simulink model "building_EXAMPLE_v1"  (R2016b)
settings: Solver=ode23tb  StartTime=-building.preruntime+8760*3600  StopTime=building.runtime+8760*3600  MaxStep=600  EnableMultiTasking=on
StartFcn:
  | tic
StopFcn:
  | toc
values from neighbouring files (symbols this model uses):
  building = create_building_automatic(building, modify, import_mode, name_XML, name_EXCEL, name_PHPP, NUMBEROFZONES)    [work_EXAMPLE_v1.m]
undefined symbols (not defined in the file or in its folder): A, B, C, cp, Dd, Dreifach, FluidMix, get_building, ID, MassFlow, p, Pressure, Qdot_C, Qdot_C_energy, Qdot_H, Qdot_H_energy, Qdot_I_electricity, Qdot_I_electricity_energy, Qdot_I_light, Qdot_I_light_energy, Qdot_I_person, Qdot_I_person_energy, Qdot_S, Qdot_S_energy, Qdot_T_ground, Qdot_T_ground_energy, Qdot_T_neighbour, Qdot_T_neighbour_energy, Qdot_T_opaque, Qdot_T_opaque_energy, Qdot_T_window, Qdot_T_window_energy, Qdot_V_infiltration, Qdot_V_infiltration_energy, Qdot_V_mech, Qdot_V_mech_energy, Qdot_V_window, Qdot_V_window_energy, rho, Tc, Temperature, Tr, Ts, Wärmeschutzglas, x_CO2, x_H2O, x_VOC
libraries: carnotUIBK x1931, carnot x83, simulink_extras x22, simulink x12
(part 4 of 35)

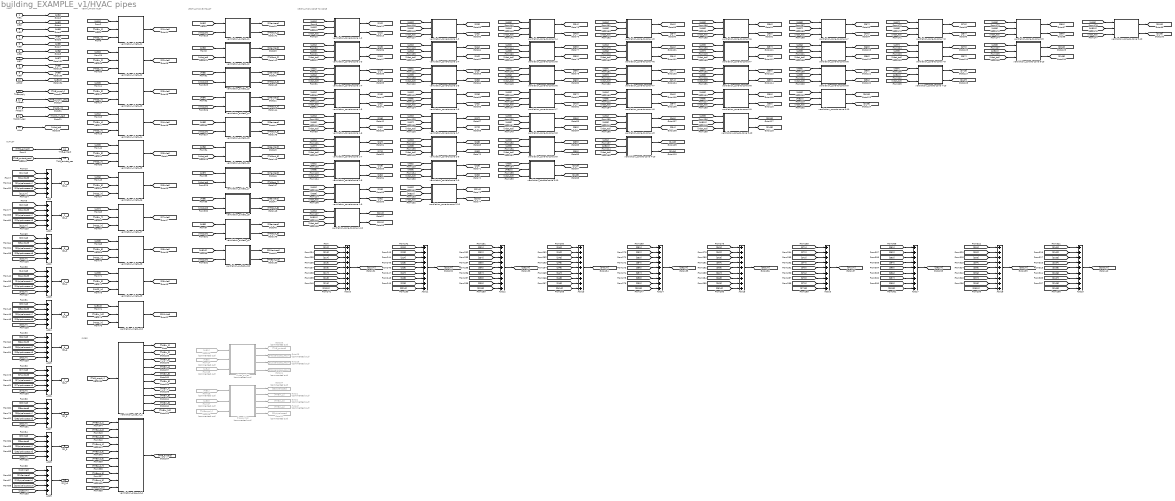
== system building_EXAMPLE_v1/HVAC pipes ==
  note: VENTILATION ZONE TO ZONE
  note: VENTILATION EXTRACT
  note: VENTILATION INLET
  note: OUTLET
  note: INLET
  note: PIPES
  AIB1 : Inport
  AIB2 : Inport  Port=2
  AIB3 : Inport  Port=3
  AIB4 : Inport  Port=4
  AIB5 : Inport  Port=5
  AIB6 : Inport  Port=6
  AIB7 : Inport  Port=7
  AIB8 : Inport  Port=8
  AIB9 : Inport  Port=9
  AIB10 : Inport  Port=10
  THBsupply : Inport  Port=11
  THBsec : Inport  Port=12
  MASSin : Inport  Port=13
  MASSin_sec : Inport  Port=14
  Vdot : Inport  Port=15
  Add{,1..9} (10 alike) : Sum  Inputs=5
  Add{10..19} (10 alike) : Sum  Inputs=9
  From23 : From  Commented=on  GotoTag=AIB1
  From24 : From  Commented=on  GotoTag=AIB3
  From25 : From  Commented=on  GotoTag=AIB4
  From26 : From  Commented=on  GotoTag=AIB1
  From27 : From  Commented=on  GotoTag=AIB3
  From28 : From  Commented=on  GotoTag=THBsupply
  Goto1 : Goto  Commented=on  GotoTag=THBin_2
  Goto2 : Goto  Commented=on  GotoTag=THBin_5
  Goto24 : Goto  Commented=on  GotoTag=S3pipelosses_return
  Goto25 : Goto  Commented=on  GotoTag=S4pipelosses_return
  Goto26 : Goto  Commented=on  GotoTag=S1pipelosses_return
  Goto27 : Goto  Commented=on  GotoTag=THBin_6
  Goto32 : Goto  Commented=on  GotoTag=S1pipelosses
  Goto33 : Goto  Commented=on  GotoTag=THB_extract
  Goto34 : Goto  Commented=on  GotoTag=S3pipelosses
  Pipes_inlet : Subsystem  Commented=on
  Pipes_outlet : Subsystem  Commented=on
  ventilation_inlet1_z1 : Subsystem  mask{perc_Vdot_tot=hvac.zone(1).inlet(1)}
  ventilation_inlet1_z10 : Subsystem  mask{perc_Vdot_tot=hvac.zone(10).inlet(1)}
  ventilation_inlet1_z2 : Subsystem  mask{perc_Vdot_tot=hvac.zone(2).inlet(1)}
  ventilation_inlet1_z3 : Subsystem  mask{perc_Vdot_tot=hvac.zone(3).inlet(1)}
  ventilation_inlet1_z4 : Subsystem  mask{perc_Vdot_tot=hvac.zone(4).inlet(1)}
  ventilation_inlet1_z5 : Subsystem  mask{perc_Vdot_tot=hvac.zone(5).inlet(1)}
  ventilation_inlet1_z6 : Subsystem  mask{perc_Vdot_tot=hvac.zone(6).inlet(1)}
  ventilation_inlet1_z7 : Subsystem  mask{perc_Vdot_tot=hvac.zone(7).inlet(1)}
  ventilation_inlet1_z8 : Subsystem  mask{perc_Vdot_tot=hvac.zone(8).inlet(1)}
  ventilation_inlet1_z9 : Subsystem  mask{perc_Vdot_tot=hvac.zone(9).inlet(1)}
  ventilation_outlet1_z1 : Subsystem  mask{perc_Vdot_tot=hvac.zone(1).outlet(1)}
  ventilation_outlet1_z10 : Subsystem  mask{perc_Vdot_tot=hvac.zone(10).outlet(1)}
  ventilation_outlet1_z2 : Subsystem  mask{perc_Vdot_tot=hvac.zone(2).outlet(1)}
  ventilation_outlet1_z3 : Subsystem  mask{perc_Vdot_tot=hvac.zone(3).outlet(1)}
  ventilation_outlet1_z4 : Subsystem  mask{perc_Vdot_tot=hvac.zone(4).outlet(1)}
  ventilation_outlet1_z5 : Subsystem  mask{perc_Vdot_tot=hvac.zone(5).outlet(1)}
  ventilation_outlet1_z6 : Subsystem  mask{perc_Vdot_tot=hvac.zone(6).outlet(1)}
  ventilation_outlet1_z7 : Subsystem  mask{perc_Vdot_tot=hvac.zone(7).outlet(1)}
  ventilation_outlet1_z8 : Subsystem  mask{perc_Vdot_tot=hvac.zone(8).outlet(1)}
  ventilation_outlet1_z9 : Subsystem  mask{perc_Vdot_tot=hvac.zone(9).outlet(1)}
  ventilation_pipe_in_1 : Subsystem
  ventilation_pipe_out_1 : Subsystem
  ventilation_zone-to-zone 1-10 : Subsystem  mask{perc_Vdot_tot=hvac.zone(1).overflow(10) - hvac.zone(10).overflow(1)}
  ventilation_zone-to-zone 1-2 : Subsystem  mask{perc_Vdot_tot=hvac.zone(1).overflow(2) - hvac.zone(2).overflow(1)}
  ventilation_zone-to-zone 1-3 : Subsystem  mask{perc_Vdot_tot=hvac.zone(1).overflow(3) - hvac.zone(3).overflow(1)}
  ventilation_zone-to-zone 1-4 : Subsystem  mask{perc_Vdot_tot=hvac.zone(1).overflow(4) - hvac.zone(4).overflow(1)}
  ventilation_zone-to-zone 1-5 : Subsystem  mask{perc_Vdot_tot=hvac.zone(1).overflow(5) - hvac.zone(5).overflow(1)}
  ventilation_zone-to-zone 1-6 : Subsystem  mask{perc_Vdot_tot=hvac.zone(1).overflow(6) - hvac.zone(6).overflow(1)}
  ventilation_zone-to-zone 1-7 : Subsystem  mask{perc_Vdot_tot=hvac.zone(1).overflow(7) - hvac.zone(7).overflow(1)}
  ventilation_zone-to-zone 1-8 : Subsystem  mask{perc_Vdot_tot=hvac.zone(1).overflow(8) - hvac.zone(8).overflow(1)}
  ventilation_zone-to-zone 1-9 : Subsystem  mask{perc_Vdot_tot=hvac.zone(1).overflow(9) - hvac.zone(9).overflow(1)}
  ventilation_zone-to-zone 2-10 : Subsystem  mask{perc_Vdot_tot=hvac.zone(2).overflow(10) - hvac.zone(10).overflow(2)}
  ventilation_zone-to-zone 2-3 : Subsystem  mask{perc_Vdot_tot=hvac.zone(2).overflow(3) - hvac.zone(3).overflow(2)}
  ventilation_zone-to-zone 2-4 : Subsystem  mask{perc_Vdot_tot=hvac.zone(2).overflow(4) - hvac.zone(4).overflow(2)}
  ventilation_zone-to-zone 2-5 : Subsystem  mask{perc_Vdot_tot=hvac.zone(2).overflow(5) - hvac.zone(5).overflow(2)}
  ventilation_zone-to-zone 2-6 : Subsystem  mask{perc_Vdot_tot=hvac.zone(2).overflow(6) - hvac.zone(6).overflow(2)}
  ventilation_zone-to-zone 2-7 : Subsystem  mask{perc_Vdot_tot=hvac.zone(2).overflow(7) - hvac.zone(7).overflow(2)}
  ventilation_zone-to-zone 2-8 : Subsystem  mask{perc_Vdot_tot=hvac.zone(2).overflow(8) - hvac.zone(8).overflow(2)}
  ventilation_zone-to-zone 2-9 : Subsystem  mask{perc_Vdot_tot=hvac.zone(2).overflow(9) - hvac.zone(9).overflow(2)}
  ventilation_zone-to-zone 3-10 : Subsystem  mask{perc_Vdot_tot=hvac.zone(3).overflow(10) - hvac.zone(10).overflow(3)}
  ventilation_zone-to-zone 3-4 : Subsystem  mask{perc_Vdot_tot=hvac.zone(3).overflow(4) - hvac.zone(4).overflow(3)}
  ventilation_zone-to-zone 3-5 : Subsystem  mask{perc_Vdot_tot=hvac.zone(3).overflow(5) - hvac.zone(5).overflow(3)}
  ventilation_zone-to-zone 3-6 : Subsystem  mask{perc_Vdot_tot=hvac.zone(3).overflow(6) - hvac.zone(6).overflow(3)}
  ventilation_zone-to-zone 3-7 : Subsystem  mask{perc_Vdot_tot=hvac.zone(3).overflow(7) - hvac.zone(7).overflow(3)}
  ventilation_zone-to-zone 3-8 : Subsystem  mask{perc_Vdot_tot=hvac.zone(3).overflow(8) - hvac.zone(8).overflow(3)}
  ventilation_zone-to-zone 3-9 : Subsystem  mask{perc_Vdot_tot=hvac.zone(3).overflow(9) - hvac.zone(9).overflow(3)}
  ventilation_zone-to-zone 4-10 : Subsystem  mask{perc_Vdot_tot=hvac.zone(4).overflow(10) - hvac.zone(10).overflow(4)}
  ventilation_zone-to-zone 4-5 : Subsystem  mask{perc_Vdot_tot=hvac.zone(4).overflow(5) - hvac.zone(5).overflow(4)}
  ventilation_zone-to-zone 4-6 : Subsystem  mask{perc_Vdot_tot=hvac.zone(4).overflow(6) - hvac.zone(6).overflow(4)}
  ventilation_zone-to-zone 4-7 : Subsystem  mask{perc_Vdot_tot=hvac.zone(4).overflow(7) - hvac.zone(7).overflow(4)}
  ventilation_zone-to-zone 4-8 : Subsystem  mask{perc_Vdot_tot=hvac.zone(4).overflow(8) - hvac.zone(8).overflow(4)}
  ventilation_zone-to-zone 4-9 : Subsystem  mask{perc_Vdot_tot=hvac.zone(4).overflow(9) - hvac.zone(9).overflow(4)}
  ventilation_zone-to-zone 5-10 : Subsystem  mask{perc_Vdot_tot=hvac.zone(5).overflow(10) - hvac.zone(10).overflow(5)}
  ventilation_zone-to-zone 5-6 : Subsystem  mask{perc_Vdot_tot=hvac.zone(5).overflow(6) - hvac.zone(6).overflow(5)}
  ventilation_zone-to-zone 5-7 : Subsystem  mask{perc_Vdot_tot=hvac.zone(5).overflow(7) - hvac.zone(7).overflow(5)}
  ventilation_zone-to-zone 5-8 : Subsystem  mask{perc_Vdot_tot=hvac.zone(5).overflow(8) - hvac.zone(8).overflow(5)}
  ventilation_zone-to-zone 5-9 : Subsystem  mask{perc_Vdot_tot=hvac.zone(5).overflow(9) - hvac.zone(9).overflow(5)}
  ventilation_zone-to-zone 6-10 : Subsystem  mask{perc_Vdot_tot=hvac.zone(6).overflow(10) - hvac.zone(10).overflow(6)}
  ventilation_zone-to-zone 6-7 : Subsystem  mask{perc_Vdot_tot=hvac.zone(6).overflow(7) - hvac.zone(7).overflow(6)}
  ventilation_zone-to-zone 6-8 : Subsystem  mask{perc_Vdot_tot=hvac.zone(6).overflow(8) - hvac.zone(8).overflow(6)}
  ventilation_zone-to-zone 6-9 : Subsystem  mask{perc_Vdot_tot=hvac.zone(6).overflow(9) - hvac.zone(9).overflow(6)}
  ventilation_zone-to-zone 7-10 : Subsystem  mask{perc_Vdot_tot=hvac.zone(7).overflow(10) - hvac.zone(10).overflow(7)}
  ventilation_zone-to-zone 7-8 : Subsystem  mask{perc_Vdot_tot=hvac.zone(7).overflow(8) - hvac.zone(8).overflow(7)}
  ventilation_zone-to-zone 7-9 : Subsystem  mask{perc_Vdot_tot=hvac.zone(7).overflow(9) - hvac.zone(9).overflow(7)}
  ventilation_zone-to-zone 8-10 : Subsystem  mask{perc_Vdot_tot=hvac.zone(8).overflow(10) - hvac.zone(10).overflow(8)}
  ventilation_zone-to-zone 8-9 : Subsystem  mask{perc_Vdot_tot=hvac.zone(8).overflow(9) - hvac.zone(9).overflow(8)}
  ventilation_zone-to-zone 9-10 : Subsystem  mask{perc_Vdot_tot=hvac.zone(9).overflow(10) - hvac.zone(10).overflow(9)}
  "[S]_1" : Outport
  "[S]_2" : Outport  Port=2
  "[S]_3" : Outport  Port=3
  "[S]_4" : Outport  Port=4
  "[S]_5" : Outport  Port=5
  "[S]_6" : Outport  Port=6
  "[S]_7" : Outport  Port=7
  "[S]_8" : Outport  Port=8
  "[S]_9" : Outport  Port=9
  "[S]_10" : Outport  Port=10
  THB_extract : Outport  Port=11
  THB_extract_sec : Outport  Port=12
  wires:
  AIB1/1 -> [AIB1]
  AIB2/1 -> [AIB2]
  AIB3/1 -> [AIB3]
  AIB4/1 -> [AIB4]
  AIB5/1 -> [AIB5]
  AIB6/1 -> [AIB6]
  [AIB1] -> ventilation_outlet1_z1/1("[AIB]")
  [AIB2] -> ventilation_inlet1_z2/1("[AIB]")
  Add/1 -> "[S]_1"/1
  [S1inlet] -> Add/1
  [S1extract] -> Add/2
  [MASS_in] -> ventilation_inlet1_z2/3(MASSin)
  From28/1 -> Pipes_inlet/3(THBvent1)
  From26/1 -> Pipes_inlet/1(AIBkueche)
  From27/1 -> Pipes_inlet/2(AIBGang)
  [S1pipelossesin] -> Add/3
  From25/1 -> Pipes_outlet/3(AIBbad)
  From23/1 -> Pipes_outlet/1(AIBkueche)
  From24/1 -> Pipes_outlet/2(AIBGang)
  Pipes_outlet/1(THB_extract) -> Goto33/1
  [S1pipelossesout] -> Add/4
  [THBin_2] -> ventilation_inlet1_z2/2(THBin)
  Pipes_inlet/2(THB eltern) -> Goto1/1
  Pipes_inlet/3(THB kind) -> Goto2/1
  Pipes_inlet/4(THB wohnz) -> Goto27/1
  THBsupply/1 -> [THB_supply]
  MASSin/1 -> [MASS_in]
  [THB_extract] -> THB_extract/1
  ventilation_inlet1_z2/1("[S]") -> [S2inlet]
  ventilation_outlet1_z1/1("[S]") -> [S1extract]
  [THB_extract_sec] -> THB_extract_sec/1
  THBsec/1 -> [THB_supply_sec]
  MASSin_sec/1 -> [MASS_in_sec]
  Pipes_outlet/3(S Kueche) -> Goto26/1
  Pipes_outlet/2(S Bad) -> Goto25/1
  Pipes_inlet/1(S Gang) -> Goto34/1
  Pipes_inlet/5(S Kueche) -> Goto32/1
  Pipes_outlet/4(S Gang) -> Goto24/1
  [AIB1] -> ventilation_inlet1_z1/1("[AIB]")
  [MASS_in] -> ventilation_inlet1_z1/3(MASSin)
  [THBin_1] -> ventilation_inlet1_z1/2(THBin)
  ventilation_inlet1_z1/1("[S]") -> [S1inlet]
  [AIB3] -> ventilation_inlet1_z3/1("[AIB]")
  [MASS_in] -> ventilation_inlet1_z3/3(MASSin)
  [THBin_3] -> ventilation_inlet1_z3/2(THBin)
  ventilation_inlet1_z3/1("[S]") -> [S3inlet]
  [AIB4] -> ventilation_inlet1_z4/1("[AIB]")
  [MASS_in] -> ventilation_inlet1_z4/3(MASSin)
  [THBin_4] -> ventilation_inlet1_z4/2(THBin)
  ventilation_inlet1_z4/1("[S]") -> [S4inlet]
  [AIB5] -> ventilation_inlet1_z5/1("[AIB]")
  [THBin_5] -> ventilation_inlet1_z5/2(THBin)
  [MASS_in] -> ventilation_inlet1_z5/3(MASSin)
  [AIB6] -> ventilation_inlet1_z6/1("[AIB]")
  [THBin_6] -> ventilation_inlet1_z6/2(THBin)
  [MASS_in] -> ventilation_inlet1_z6/3(MASSin)
  ventilation_inlet1_z5/1("[S]") -> [S5inlet]
  ventilation_inlet1_z6/1("[S]") -> [S6inlet]
  [AIB7] -> ventilation_inlet1_z7/1("[AIB]")
  [THBin_7] -> ventilation_inlet1_z7/2(THBin)
  [MASS_in] -> ventilation_inlet1_z7/3(MASSin)
  ventilation_inlet1_z7/1("[S]") -> [S7inlet]
  [AIB8] -> ventilation_inlet1_z8/1("[AIB]")
  [THBin_8] -> ventilation_inlet1_z8/2(THBin)
  [MASS_in] -> ventilation_inlet1_z8/3(MASSin)
  ventilation_inlet1_z8/1("[S]") -> [S8inlet]
  [AIB9] -> ventilation_inlet1_z9/1("[AIB]")
  [THBin_9] -> ventilation_inlet1_z9/2(THBin)
  [MASS_in] -> ventilation_inlet1_z9/3(MASSin)
  ventilation_inlet1_z9/1("[S]") -> [S9inlet]
  [AIB10] -> ventilation_inlet1_z10/1("[AIB]")
  [THBin_10] -> ventilation_inlet1_z10/2(THBin)
  [MASS_in] -> ventilation_inlet1_z10/3(MASSin)
  ventilation_inlet1_z10/1("[S]") -> [S10inlet]
  Add1/1 -> "[S]_2"/1
  [S2inlet] -> Add1/1
  [S2extract] -> Add1/2
  [S2pipelossesin] -> Add1/3
  [S2pipelossesout] -> Add1/4
  Add2/1 -> "[S]_3"/1
  [S3inlet] -> Add2/1
  [S3extract] -> Add2/2
  [S3pipelossesin] -> Add2/3
  [S3pipelossesout] -> Add2/4
  Add3/1 -> "[S]_4"/1
  [S4inlet] -> Add3/1
  [S4extract] -> Add3/2
  [S4pipelossesin] -> Add3/3
  [S4pipelossesout] -> Add3/4
  Add4/1 -> "[S]_5"/1
  [S5inlet] -> Add4/1
  [S5extract] -> Add4/2
  [S5pipelossesin] -> Add4/3
  [S5pipelossesout] -> Add4/4
  Add5/1 -> "[S]_6"/1
  [S6inlet] -> Add5/1
  [S6extract] -> Add5/2
  [S6pipelossesin] -> Add5/3
  [S6pipelossesout] -> Add5/4
  Add6/1 -> "[S]_7"/1
  [S7inlet] -> Add6/1
  [S7extract] -> Add6/2
  [S7pipelossesin] -> Add6/3
  [S7pipelossesout] -> Add6/4
  Add7/1 -> "[S]_8"/1
  [S8inlet] -> Add7/1
  [S8extract] -> Add7/2
  [S8pipelossesin] -> Add7/3
  [S8pipelossesout] -> Add7/4
  Add8/1 -> "[S]_9"/1
  [S9inlet] -> Add8/1
  [S9extract] -> Add8/2
  [S9pipelossesin] -> Add8/3
  [S9pipelossesout] -> Add8/4
  Add9/1 -> "[S]_10"/1
  [S10inlet] -> Add9/1
  [S10extract] -> Add9/2
  [S10pipelossesin] -> Add9/3
  [S10pipelossesout] -> Add9/4
  ventilation_outlet1_z2/1("[S]") -> [S2extract]
  ventilation_outlet1_z3/1("[S]") -> [S3extract]
  ventilation_outlet1_z4/1("[S]") -> [S4extract]
  [AIB2] -> ventilation_outlet1_z2/1("[AIB]")
  [AIB3] -> ventilation_outlet1_z3/1("[AIB]")
  [AIB4] -> ventilation_outlet1_z4/1("[AIB]")
  ventilation_outlet1_z5/1("[S]") -> [S5extract]
  ventilation_outlet1_z6/1("[S]") -> [S6extract]
  ventilation_outlet1_z7/1("[S]") -> [S7extract]
  ventilation_outlet1_z8/1("[S]") -> [S8extract]
  ventilation_outlet1_z9/1("[S]") -> [S9extract]
  ventilation_outlet1_z10/1("[S]") -> [S10extract]
  [AIB5] -> ventilation_outlet1_z5/1("[AIB]")
  [AIB6] -> ventilation_outlet1_z6/1("[AIB]")
  [AIB7] -> ventilation_outlet1_z7/1("[AIB]")
  [AIB8] -> ventilation_outlet1_z8/1("[AIB]")
  [AIB9] -> ventilation_outlet1_z9/1("[AIB]")
  [AIB10] -> ventilation_outlet1_z10/1("[AIB]")
  [AIB1] -> ventilation_zone-to-zone 1-2/1("[AIB]_in")
  [AIB2] -> ventilation_zone-to-zone 1-2/2("[AIB]_out")
  ventilation_zone-to-zone 1-2/1("[S]_in") -> [S12]
  ventilation_zone-to-zone 1-2/2("[S]_out") -> [S21]
  [Vdot_tot] -> ventilation_zone-to-zone 1-2/3(Vdot)
  [AIB1] -> ventilation_zone-to-zone 1-3/1("[AIB]_in")
  [AIB3] -> ventilation_zone-to-zone 1-3/2("[AIB]_out")
  ventilation_zone-to-zone 1-3/1("[S]_in") -> [S13]
  ventilation_zone-to-zone 1-3/2("[S]_out") -> [S31]
  [Vdot_tot] -> ventilation_zone-to-zone 1-3/3(Vdot)
  [AIB1] -> ventilation_zone-to-zone 1-4/1("[AIB]_in")
  ventilation_zone-to-zone 1-4/1("[S]_in") -> [S14]
  ventilation_zone-to-zone 1-4/2("[S]_out") -> [S41]
  [Vdot_tot] -> ventilation_zone-to-zone 1-4/3(Vdot)
  [AIB1] -> ventilation_zone-to-zone 1-5/1("[AIB]_in")
  ventilation_zone-to-zone 1-5/1("[S]_in") -> [S15]
  ventilation_zone-to-zone 1-5/2("[S]_out") -> [S51]
  [Vdot_tot] -> ventilation_zone-to-zone 1-5/3(Vdot)
  [AIB1] -> ventilation_zone-to-zone 1-6/1("[AIB]_in")
  ventilation_zone-to-zone 1-6/1("[S]_in") -> [S16]
  ventilation_zone-to-zone 1-6/2("[S]_out") -> [S61]
  [Vdot_tot] -> ventilation_zone-to-zone 1-6/3(Vdot)
  [AIB1] -> ventilation_zone-to-zone 1-7/1("[AIB]_in")
  ventilation_zone-to-zone 1-7/1("[S]_in") -> [S17]
  ventilation_zone-to-zone 1-7/2("[S]_out") -> [S71]
  [Vdot_tot] -> ventilation_zone-to-zone 1-7/3(Vdot)
  [AIB1] -> ventilation_zone-to-zone 1-8/1("[AIB]_in")
  ventilation_zone-to-zone 1-8/1("[S]_in") -> [S18]
  ventilation_zone-to-zone 1-8/2("[S]_out") -> [S81]
  [Vdot_tot] -> ventilation_zone-to-zone 1-8/3(Vdot)
  [AIB1] -> ventilation_zone-to-zone 1-9/1("[AIB]_in")
  ventilation_zone-to-zone 1-9/1("[S]_in") -> [S19]
  ventilation_zone-to-zone 1-9/2("[S]_out") -> [S91]
  [Vdot_tot] -> ventilation_zone-to-zone 1-9/3(Vdot)
  [AIB1] -> ventilation_zone-to-zone 1-10/1("[AIB]_in")
  ventilation_zone-to-zone 1-10/1("[S]_in") -> [S110]
  ventilation_zone-to-zone 1-10/2("[S]_out") -> [S101]
  [Vdot_tot] -> ventilation_zone-to-zone 1-10/3(Vdot)
  [AIB4] -> ventilation_zone-to-zone 1-4/2("[AIB]_out")
  [AIB5] -> ventilation_zone-to-zone 1-5/2("[AIB]_out")
  [AIB6] -> ventilation_zone-to-zone 1-6/2("[AIB]_out")
  [AIB7] -> ventilation_zone-to-zone 1-7/2("[AIB]_out")
  [AIB8] -> ventilation_zone-to-zone 1-8/2("[AIB]_out")
  [AIB9] -> ventilation_zone-to-zone 1-9/2("[AIB]_out")
  [AIB10] -> ventilation_zone-to-zone 1-10/2("[AIB]_out")
  [AIB2] -> ventilation_zone-to-zone 2-3/1("[AIB]_in")
  [AIB3] -> ventilation_zone-to-zone 2-3/2("[AIB]_out")
  ventilation_zone-to-zone 2-3/1("[S]_in") -> [S23]
  ventilation_zone-to-zone 2-3/2("[S]_out") -> [S32]
  [Vdot_tot] -> ventilation_zone-to-zone 2-3/3(Vdot)
  [AIB2] -> ventilation_zone-to-zone 2-4/1("[AIB]_in")
  [AIB4] -> ventilation_zone-to-zone 2-4/2("[AIB]_out")
  ventilation_zone-to-zone 2-4/1("[S]_in") -> [S24]
  ventilation_zone-to-zone 2-4/2("[S]_out") -> [S42]
  [Vdot_tot] -> ventilation_zone-to-zone 2-4/3(Vdot)
  [AIB2] -> ventilation_zone-to-zone 2-5/1("[AIB]_in")
  [AIB5] -> ventilation_zone-to-zone 2-5/2("[AIB]_out")
  ventilation_zone-to-zone 2-5/1("[S]_in") -> [S25]
  ventilation_zone-to-zone 2-5/2("[S]_out") -> [S52]
  [Vdot_tot] -> ventilation_zone-to-zone 2-5/3(Vdot)
  [AIB2] -> ventilation_zone-to-zone 2-6/1("[AIB]_in")
  [AIB6] -> ventilation_zone-to-zone 2-6/2("[AIB]_out")
  ventilation_zone-to-zone 2-6/1("[S]_in") -> [S26]
  ventilation_zone-to-zone 2-6/2("[S]_out") -> [S62]
  [Vdot_tot] -> ventilation_zone-to-zone 2-6/3(Vdot)
  [AIB2] -> ventilation_zone-to-zone 2-7/1("[AIB]_in")
  [AIB7] -> ventilation_zone-to-zone 2-7/2("[AIB]_out")
  ventilation_zone-to-zone 2-7/1("[S]_in") -> [S27]
  ventilation_zone-to-zone 2-7/2("[S]_out") -> [S72]
  [Vdot_tot] -> ventilation_zone-to-zone 2-7/3(Vdot)
  [AIB2] -> ventilation_zone-to-zone 2-8/1("[AIB]_in")
  [AIB8] -> ventilation_zone-to-zone 2-8/2("[AIB]_out")
  ventilation_zone-to-zone 2-8/1("[S]_in") -> [S28]
  ventilation_zone-to-zone 2-8/2("[S]_out") -> [S82]
  [Vdot_tot] -> ventilation_zone-to-zone 2-8/3(Vdot)
  [AIB2] -> ventilation_zone-to-zone 2-9/1("[AIB]_in")
  [AIB9] -> ventilation_zone-to-zone 2-9/2("[AIB]_out")
  ventilation_zone-to-zone 2-9/1("[S]_in") -> [S29]
  ventilation_zone-to-zone 2-9/2("[S]_out") -> [S92]
  [Vdot_tot] -> ventilation_zone-to-zone 2-9/3(Vdot)
  [AIB2] -> ventilation_zone-to-zone 2-10/1("[AIB]_in")
  [AIB10] -> ventilation_zone-to-zone 2-10/2("[AIB]_out")
  ventilation_zone-to-zone 2-10/1("[S]_in") -> [S210]
  ventilation_zone-to-zone 2-10/2("[S]_out") -> [S102]
  [Vdot_tot] -> ventilation_zone-to-zone 2-10/3(Vdot)
  [AIB3] -> ventilation_zone-to-zone 3-4/1("[AIB]_in")
  [AIB4] -> ventilation_zone-to-zone 3-4/2("[AIB]_out")
  ventilation_zone-to-zone 3-4/1("[S]_in") -> [S34]
  ventilation_zone-to-zone 3-4/2("[S]_out") -> [S43]
  [Vdot_tot] -> ventilation_zone-to-zone 3-4/3(Vdot)
  [AIB3] -> ventilation_zone-to-zone 3-5/1("[AIB]_in")
  [AIB5] -> ventilation_zone-to-zone 3-5/2("[AIB]_out")
  ventilation_zone-to-zone 3-5/1("[S]_in") -> [S35]
  ventilation_zone-to-zone 3-5/2("[S]_out") -> [S53]
  [Vdot_tot] -> ventilation_zone-to-zone 3-5/3(Vdot)
  [AIB3] -> ventilation_zone-to-zone 3-6/1("[AIB]_in")
  [AIB6] -> ventilation_zone-to-zone 3-6/2("[AIB]_out")
  ventilation_zone-to-zone 3-6/1("[S]_in") -> [S36]
  ventilation_zone-to-zone 3-6/2("[S]_out") -> [S63]
  [Vdot_tot] -> ventilation_zone-to-zone 3-6/3(Vdot)
  [AIB3] -> ventilation_zone-to-zone 3-7/1("[AIB]_in")
  [AIB7] -> ventilation_zone-to-zone 3-7/2("[AIB]_out")
  ventilation_zone-to-zone 3-7/1("[S]_in") -> [S37]
  ventilation_zone-to-zone 3-7/2("[S]_out") -> [S73]
  [Vdot_tot] -> ventilation_zone-to-zone 3-7/3(Vdot)
  [AIB3] -> ventilation_zone-to-zone 3-8/1("[AIB]_in")
  [AIB8] -> ventilation_zone-to-zone 3-8/2("[AIB]_out")
  ventilation_zone-to-zone 3-8/1("[S]_in") -> [S38]
  ventilation_zone-to-zone 3-8/2("[S]_out") -> [S83]
  [Vdot_tot] -> ventilation_zone-to-zone 3-8/3(Vdot)
  [AIB3] -> ventilation_zone-to-zone 3-9/1("[AIB]_in")
  [AIB9] -> ventilation_zone-to-zone 3-9/2("[AIB]_out")
  ventilation_zone-to-zone 3-9/1("[S]_in") -> [S39]
  ventilation_zone-to-zone 3-9/2("[S]_out") -> [S93]
  [Vdot_tot] -> ventilation_zone-to-zone 3-9/3(Vdot)
  [AIB3] -> ventilation_zone-to-zone 3-10/1("[AIB]_in")
  [AIB10] -> ventilation_zone-to-zone 3-10/2("[AIB]_out")
  ventilation_zone-to-zone 3-10/1("[S]_in") -> [S310]
  ventilation_zone-to-zone 3-10/2("[S]_out") -> [S103]
  [Vdot_tot] -> ventilation_zone-to-zone 3-10/3(Vdot)
  [AIB4] -> ventilation_zone-to-zone 4-5/1("[AIB]_in")
  [AIB5] -> ventilation_zone-to-zone 4-5/2("[AIB]_out")
  ventilation_zone-to-zone 4-5/1("[S]_in") -> [S45]
  ventilation_zone-to-zone 4-5/2("[S]_out") -> [S54]
  [Vdot_tot] -> ventilation_zone-to-zone 4-5/3(Vdot)
  [AIB5] -> ventilation_zone-to-zone 5-6/1("[AIB]_in")
  [AIB6] -> ventilation_zone-to-zone 5-6/2("[AIB]_out")
  ventilation_zone-to-zone 5-6/1("[S]_in") -> [S56]
  ventilation_zone-to-zone 5-6/2("[S]_out") -> [S65]
  [Vdot_tot] -> ventilation_zone-to-zone 5-6/3(Vdot)
  [AIB6] -> ventilation_zone-to-zone 6-7/1("[AIB]_in")
  [AIB7] -> ventilation_zone-to-zone 6-7/2("[AIB]_out")
  ventilation_zone-to-zone 6-7/1("[S]_in") -> [S67]
  ventilation_zone-to-zone 6-7/2("[S]_out") -> [S76]
  [Vdot_tot] -> ventilation_zone-to-zone 6-7/3(Vdot)
  [AIB7] -> ventilation_zone-to-zone 7-8/1("[AIB]_in")
  [AIB8] -> ventilation_zone-to-zone 7-8/2("[AIB]_out")
  ventilation_zone-to-zone 7-8/1("[S]_in") -> [S78]
  ventilation_zone-to-zone 7-8/2("[S]_out") -> [S87]
  [Vdot_tot] -> ventilation_zone-to-zone 7-8/3(Vdot)
  [AIB8] -> ventilation_zone-to-zone 8-9/1("[AIB]_in")
  [AIB9] -> ventilation_zone-to-zone 8-9/2("[AIB]_out")
  ventilation_zone-to-zone 8-9/1("[S]_in") -> [S89]
  ventilation_zone-to-zone 8-9/2("[S]_out") -> [S98]
  [Vdot_tot] -> ventilation_zone-to-zone 8-9/3(Vdot)
  [AIB9] -> ventilation_zone-to-zone 9-10/1("[AIB]_in")
  [AIB10] -> ventilation_zone-to-zone 9-10/2("[AIB]_out")
  ventilation_zone-to-zone 9-10/1("[S]_in") -> [S910]
  ventilation_zone-to-zone 9-10/2("[S]_out") -> [S109]
  [Vdot_tot] -> ventilation_zone-to-zone 9-10/3(Vdot)
  [AIB4] -> ventilation_zone-to-zone 4-6/1("[AIB]_in")
  [AIB6] -> ventilation_zone-to-zone 4-6/2("[AIB]_out")
  ventilation_zone-to-zone 4-6/1("[S]_in") -> [S46]
  ventilation_zone-to-zone 4-6/2("[S]_out") -> [S64]
  [Vdot_tot] -> ventilation_zone-to-zone 4-6/3(Vdot)
  [AIB4] -> ventilation_zone-to-zone 4-7/1("[AIB]_in")
  [AIB7] -> ventilation_zone-to-zone 4-7/2("[AIB]_out")
  ventilation_zone-to-zone 4-7/1("[S]_in") -> [S47]
  ventilation_zone-to-zone 4-7/2("[S]_out") -> [S74]
  [Vdot_tot] -> ventilation_zone-to-zone 4-7/3(Vdot)
  [AIB4] -> ventilation_zone-to-zone 4-8/1("[AIB]_in")
  [AIB8] -> ventilation_zone-to-zone 4-8/2("[AIB]_out")
  ventilation_zone-to-zone 4-8/1("[S]_in") -> [S48]
  ventilation_zone-to-zone 4-8/2("[S]_out") -> [S84]
  [Vdot_tot] -> ventilation_zone-to-zone 4-8/3(Vdot)
  [AIB4] -> ventilation_zone-to-zone 4-9/1("[AIB]_in")
  [AIB9] -> ventilation_zone-to-zone 4-9/2("[AIB]_out")
  ventilation_zone-to-zone 4-9/1("[S]_in") -> [S49]
  ventilation_zone-to-zone 4-9/2("[S]_out") -> [S94]
  [Vdot_tot] -> ventilation_zone-to-zone 4-9/3(Vdot)
  [AIB4] -> ventilation_zone-to-zone 4-10/1("[AIB]_in")
  [AIB10] -> ventilation_zone-to-zone 4-10/2("[AIB]_out")
  ventilation_zone-to-zone 4-10/1("[S]_in") -> [S410]
  ventilation_zone-to-zone 4-10/2("[S]_out") -> [S104]
  [Vdot_tot] -> ventilation_zone-to-zone 4-10/3(Vdot)
  [AIB5] -> ventilation_zone-to-zone 5-7/1("[AIB]_in")
  [AIB7] -> ventilation_zone-to-zone 5-7/2("[AIB]_out")
  ventilation_zone-to-zone 5-7/1("[S]_in") -> [S57]
  ventilation_zone-to-zone 5-7/2("[S]_out") -> [S75]
  [Vdot_tot] -> ventilation_zone-to-zone 5-7/3(Vdot)
  [AIB5] -> ventilation_zone-to-zone 5-8/1("[AIB]_in")
  [AIB8] -> ventilation_zone-to-zone 5-8/2("[AIB]_out")
  ventilation_zone-to-zone 5-8/1("[S]_in") -> [S58]
  ventilation_zone-to-zone 5-8/2("[S]_out") -> [S85]
  [Vdot_tot] -> ventilation_zone-to-zone 5-8/3(Vdot)
  [AIB5] -> ventilation_zone-to-zone 5-9/1("[AIB]_in")
  [AIB9] -> ventilation_zone-to-zone 5-9/2("[AIB]_out")
  ventilation_zone-to-zone 5-9/1("[S]_in") -> [S59]
  ventilation_zone-to-zone 5-9/2("[S]_out") -> [S95]
  [Vdot_tot] -> ventilation_zone-to-zone 5-9/3(Vdot)
  [AIB5] -> ventilation_zone-to-zone 5-10/1("[AIB]_in")
  [AIB10] -> ventilation_zone-to-zone 5-10/2("[AIB]_out")
  ventilation_zone-to-zone 5-10/1("[S]_in") -> [S510]
  ventilation_zone-to-zone 5-10/2("[S]_out") -> [S105]
  [Vdot_tot] -> ventilation_zone-to-zone 5-10/3(Vdot)
  [AIB6] -> ventilation_zone-to-zone 6-8/1("[AIB]_in")
  [AIB8] -> ventilation_zone-to-zone 6-8/2("[AIB]_out")
  ventilation_zone-to-zone 6-8/1("[S]_in") -> [S68]
  ventilation_zone-to-zone 6-8/2("[S]_out") -> [S86]
  [Vdot_tot] -> ventilation_zone-to-zone 6-8/3(Vdot)
  [AIB6] -> ventilation_zone-to-zone 6-9/1("[AIB]_in")
  [AIB9] -> ventilation_zone-to-zone 6-9/2("[AIB]_out")
  ventilation_zone-to-zone 6-9/1("[S]_in") -> [S69]
  ventilation_zone-to-zone 6-9/2("[S]_out") -> [S96]
  [Vdot_tot] -> ventilation_zone-to-zone 6-9/3(Vdot)
  [AIB6] -> ventilation_zone-to-zone 6-10/1("[AIB]_in")
  [AIB10] -> ventilation_zone-to-zone 6-10/2("[AIB]_out")
  ventilation_zone-to-zone 6-10/1("[S]_in") -> [S610]
  ventilation_zone-to-zone 6-10/2("[S]_out") -> [S106]
  [Vdot_tot] -> ventilation_zone-to-zone 6-10/3(Vdot)
  [AIB7] -> ventilation_zone-to-zone 7-9/1("[AIB]_in")
  [AIB9] -> ventilation_zone-to-zone 7-9/2("[AIB]_out")
  ventilation_zone-to-zone 7-9/1("[S]_in") -> [S79]
  ventilation_zone-to-zone 7-9/2("[S]_out") -> [S97]
  [Vdot_tot] -> ventilation_zone-to-zone 7-9/3(Vdot)
  [AIB7] -> ventilation_zone-to-zone 7-10/1("[AIB]_in")
  [AIB10] -> ventilation_zone-to-zone 7-10/2("[AIB]_out")
  ventilation_zone-to-zone 7-10/1("[S]_in") -> [S710]
  ventilation_zone-to-zone 7-10/2("[S]_out") -> [S107]
  [Vdot_tot] -> ventilation_zone-to-zone 7-10/3(Vdot)
  [AIB8] -> ventilation_zone-to-zone 8-10/1("[AIB]_in")
  [AIB10] -> ventilation_zone-to-zone 8-10/2("[AIB]_out")
  ventilation_zone-to-zone 8-10/1("[S]_in") -> [S810]
  ventilation_zone-to-zone 8-10/2("[S]_out") -> [S108]
  [Vdot_tot] -> ventilation_zone-to-zone 8-10/3(Vdot)
  [S12] -> Add10/1
  Add10/1 -> [S1sum]
  [S1sum] -> Add/5
  [S2sum] -> Add1/5
  [S3sum] -> Add2/5
  [S4sum] -> Add3/5
  [S5sum] -> Add4/5
  [S6sum] -> Add5/5
  [S7sum] -> Add6/5
  [S8sum] -> Add7/5
  [S9sum] -> Add8/5
  [S10sum] -> Add9/5
  Add11/1 -> [S2sum]
  Add12/1 -> [S3sum]
  Add13/1 -> [S4sum]
  Add14/1 -> [S5sum]
  Add15/1 -> [S6sum]
  Add16/1 -> [S7sum]
  Add17/1 -> [S8sum]
  Add18/1 -> [S9sum]
  Add19/1 -> [S10sum]
  [S13] -> Add10/2
  [S15] -> Add10/4
  [S14] -> Add10/3
  [S16] -> Add10/5
  [S17] -> Add10/6
  [S18] -> Add10/7
  [S19] -> Add10/8
  [S110] -> Add10/9
  [S21] -> Add11/1
  [S23] -> Add11/2
  [S24] -> Add11/3
  [S25] -> Add11/4
  [S26] -> Add11/5
  [S27] -> Add11/6
  [S28] -> Add11/7
  [S29] -> Add11/8
  [S210] -> Add11/9
  [S31] -> Add12/1
  [S32] -> Add12/2
  [S34] -> Add12/3
  [S35] -> Add12/4
  [S36] -> Add12/5
  [S37] -> Add12/6
  [S38] -> Add12/7
  [S39] -> Add12/8
  [S310] -> Add12/9
  [S41] -> Add13/1
  [S42] -> Add13/2
  [S43] -> Add13/3
  [S45] -> Add13/4
  [S46] -> Add13/5
  [S47] -> Add13/6
  [S48] -> Add13/7
  [S49] -> Add13/8
  [S410] -> Add13/9
  [S51] -> Add14/1
  [S52] -> Add14/2
  [S53] -> Add14/3
  [S54] -> Add14/4
  [S56] -> Add14/5
  [S57] -> Add14/6
  [S58] -> Add14/7
  [S59] -> Add14/8
  [S510] -> Add14/9
  [S61] -> Add15/1
  [S62] -> Add15/2
  [S63] -> Add15/3
  [S64] -> Add15/4
  [S65] -> Add15/5
  [S67] -> Add15/6
  [S68] -> Add15/7
  [S69] -> Add15/8
  [S610] -> Add15/9
  [S71] -> Add16/1
  [S72] -> Add16/2
  [S73] -> Add16/3
  [S74] -> Add16/4
  [S75] -> Add16/5
  [S76] -> Add16/6
  [S78] -> Add16/7
  [S79] -> Add16/8
  [S710] -> Add16/9
  [S81] -> Add17/1
  [S82] -> Add17/2
  [S83] -> Add17/3
  [S84] -> Add17/4
  [S85] -> Add17/5
  [S86] -> Add17/6
  [S87] -> Add17/7
  [S89] -> Add17/8
  [S810] -> Add17/9
  [S91] -> Add18/1
  [S101] -> Add19/1
  [S92] -> Add18/2
  [S93] -> Add18/3
  [S94] -> Add18/4
  [S95] -> Add18/5
  [S96] -> Add18/6
  [S97] -> Add18/7
  [S98] -> Add18/8
  [S910] -> Add18/9
  [S102] -> Add19/2
  [S103] -> Add19/3
  [S104] -> Add19/4
  [S105] -> Add19/5
  [S106] -> Add19/6
  [S107] -> Add19/7
  [S108] -> Add19/8
  [S109] -> Add19/9
  [Vdot_tot] -> ventilation_outlet1_z1/2(Vdot)
  [Vdot_tot] -> ventilation_outlet1_z2/2(Vdot)
  [Vdot_tot] -> ventilation_outlet1_z3/2(Vdot)
  [Vdot_tot] -> ventilation_outlet1_z4/2(Vdot)
  [Vdot_tot] -> ventilation_outlet1_z5/2(Vdot)
  [Vdot_tot] -> ventilation_outlet1_z6/2(Vdot)
  [Vdot_tot] -> ventilation_outlet1_z7/2(Vdot)
  [Vdot_tot] -> ventilation_outlet1_z8/2(Vdot)
  [Vdot_tot] -> ventilation_outlet1_z9/2(Vdot)
  [Vdot_tot] -> ventilation_outlet1_z10/2(Vdot)
  ventilation_outlet1_z1/2(THBout) -> [THBout_1]
  ventilation_outlet1_z2/2(THBout) -> [THBout_2]
  ventilation_outlet1_z3/2(THBout) -> [THBout_3]
  ventilation_outlet1_z4/2(THBout) -> [THBout_4]
  ventilation_outlet1_z5/2(THBout) -> [THBout_5]
  ventilation_outlet1_z6/2(THBout) -> [THBout_6]
  ventilation_outlet1_z7/2(THBout) -> [THBout_7]
  ventilation_outlet1_z8/2(THBout) -> [THBout_8]
  ventilation_outlet1_z9/2(THBout) -> [THBout_9]
  ventilation_outlet1_z10/2(THBout) -> [THBout_10]
  [THB_supply] -> ventilation_pipe_in_1/1(THBsupply)
  ventilation_pipe_in_1/1("[TVBin_1]") -> [THBin_1]
  Vdot/1 -> [Vdot_tot]
  AIB7/1 -> [AIB7]
  AIB8/1 -> [AIB8]
  AIB9/1 -> [AIB9]
  AIB10/1 -> [AIB10]
  ventilation_pipe_in_1/2("[TVBin_2]") -> [THBin_2]
  ventilation_pipe_in_1/3("[TVBin_3]") -> [THBin_3]
  ventilation_pipe_in_1/4("[TVBin_4]") -> [THBin_4]
  ventilation_pipe_in_1/7("[TVBin_7]") -> [THBin_7]
  ventilation_pipe_in_1/6("[TVBin_6]") -> [THBin_6]
  ventilation_pipe_in_1/5("[TVBin_5]") -> [THBin_5]
  ventilation_pipe_in_1/8("[TVBin_8]") -> [THBin_8]
  ventilation_pipe_in_1/9("[TVBin_9]") -> [THBin_9]
  ventilation_pipe_in_1/10("[TVBin_10]") -> [THBin_10]
  ventilation_pipe_out_1/1(THBextract) -> [THB_extract]
  [THBout_1] -> ventilation_pipe_out_1/1("[THBout_1]")
  [THBout_2] -> ventilation_pipe_out_1/2("[THBout_2]")
  [THBout_3] -> ventilation_pipe_out_1/3("[THBout_3]")
  [THBout_4] -> ventilation_pipe_out_1/4("[THBout_4]")
  [THBout_5] -> ventilation_pipe_out_1/5("[THBout_5]")
  [THBout_6] -> ventilation_pipe_out_1/6("[THBout_6]")
  [THBout_10] -> ventilation_pipe_out_1/10("[THBout_10]")
  [THBout_8] -> ventilation_pipe_out_1/8("[THBout_8]")
  [THBout_9] -> ventilation_pipe_out_1/9("[THBout_9]")
  [THBout_7] -> ventilation_pipe_out_1/7("[THBout_7]")

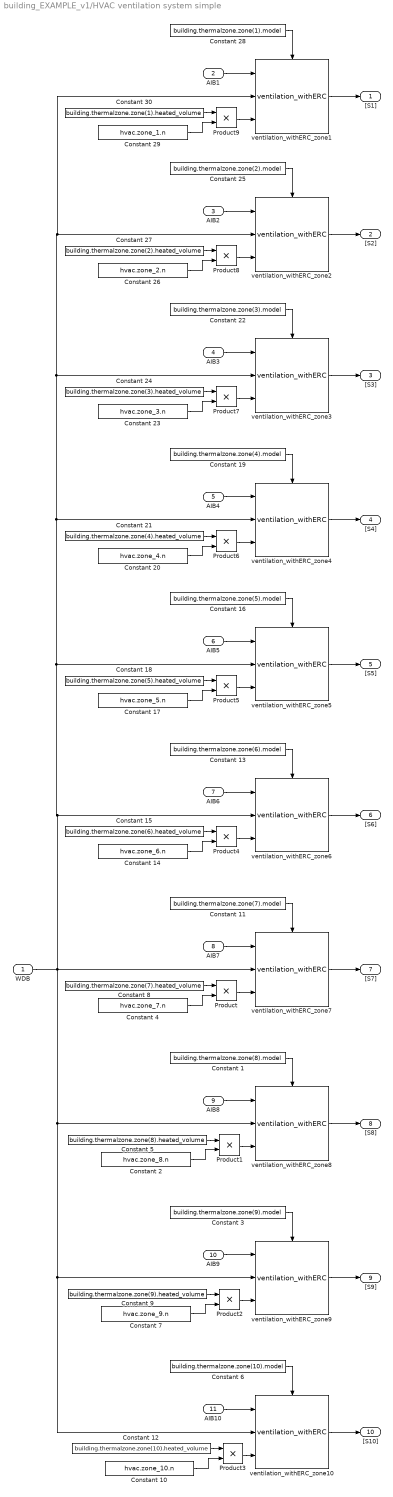
== system building_EXAMPLE_v1/HVAC ventilation system simple ==
  WDB : Inport
  AIB1 : Inport  Port=2
  AIB2 : Inport  Port=3
  AIB3 : Inport  Port=4
  AIB4 : Inport  Port=5
  AIB5 : Inport  Port=6
  AIB6 : Inport  Port=7
  AIB7 : Inport  Port=8
  "AIB8 " : Inport  Port=9
  AIB9 : Inport  Port=10
  AIB10 : Inport  Port=11
  Constant 1 : Constant  Value=building.thermalzone.zone(8).model  VectorParams1D=off
  Constant 10 : Constant  Value=hvac.zone_10.n  VectorParams1D=off
  Constant 11 : Constant  Value=building.thermalzone.zone(7).model  VectorParams1D=off
  Constant 12 : Constant  Value=building.thermalzone.zone(10).heated_volume  VectorParams1D=off
  Constant 13 : Constant  Value=building.thermalzone.zone(6).model  VectorParams1D=off
  Constant 14 : Constant  Value=hvac.zone_6.n  VectorParams1D=off
  Constant 15 : Constant  Value=building.thermalzone.zone(6).heated_volume  VectorParams1D=off
  Constant 16 : Constant  Value=building.thermalzone.zone(5).model  VectorParams1D=off
  Constant 17 : Constant  Value=hvac.zone_5.n  VectorParams1D=off
  Constant 18 : Constant  Value=building.thermalzone.zone(5).heated_volume  VectorParams1D=off
  Constant 19 : Constant  Value=building.thermalzone.zone(4).model  VectorParams1D=off
  Constant 2 : Constant  Value=hvac.zone_8.n  VectorParams1D=off
  Constant 20 : Constant  Value=hvac.zone_4.n  VectorParams1D=off
  Constant 21 : Constant  Value=building.thermalzone.zone(4).heated_volume  VectorParams1D=off
  Constant 22 : Constant  Value=building.thermalzone.zone(3).model  VectorParams1D=off
  Constant 23 : Constant  Value=hvac.zone_3.n  VectorParams1D=off
  Constant 24 : Constant  Value=building.thermalzone.zone(3).heated_volume  VectorParams1D=off
  Constant 25 : Constant  Value=building.thermalzone.zone(2).model  VectorParams1D=off
  Constant 26 : Constant  Value=hvac.zone_2.n  VectorParams1D=off
  Constant 27 : Constant  Value=building.thermalzone.zone(2).heated_volume  VectorParams1D=off
  Constant 28 : Constant  Value=building.thermalzone.zone(1).model  VectorParams1D=off
  Constant 29 : Constant  Value=hvac.zone_1.n  VectorParams1D=off
  Constant 3 : Constant  Value=building.thermalzone.zone(9).model  VectorParams1D=off
  Constant 30 : Constant  Value=building.thermalzone.zone(1).heated_volume  VectorParams1D=off
  Constant 4 : Constant  Value=hvac.zone_7.n  VectorParams1D=off
  Constant 5 : Constant  Value=building.thermalzone.zone(8).heated_volume  VectorParams1D=off
  Constant 6 : Constant  Value=building.thermalzone.zone(10).model  VectorParams1D=off
  Constant 7 : Constant  Value=hvac.zone_9.n  VectorParams1D=off
  Constant 8 : Constant  Value=building.thermalzone.zone(7).heated_volume  VectorParams1D=off
  Constant 9 : Constant  Value=building.thermalzone.zone(9).heated_volume  VectorParams1D=off
  Product{,1..9} (10 alike) : Product
  ventilation_withERC_zone{1..10} (10 alike) : carnotUIBK/HVAC/ventilation_withERC  co2=400  eta=hvac.eta  eta_x=hvac.eta_x
  "[S1]" : Outport
  "[S2]" : Outport  Port=2
  "[S3]" : Outport  Port=3
  "[S4]" : Outport  Port=4
  "[S5]" : Outport  Port=5
  "[S6]" : Outport  Port=6
  "[S7]" : Outport  Port=7
  "[S8]" : Outport  Port=8
  "[S9]" : Outport  Port=9
  "[S10]" : Outport  Port=10
  wires:
  AIB7/1 -> ventilation_withERC_zone7/1
  ventilation_withERC_zone7/1 -> "[S7]"/1
  Constant 11/1 -> ventilation_withERC_zone7/Enable
  "AIB8 "/1 -> ventilation_withERC_zone8/1
  Product1/1 -> ventilation_withERC_zone8/3
  ventilation_withERC_zone8/1 -> "[S8]"/1
  Constant 1/1 -> ventilation_withERC_zone8/Enable
  AIB9/1 -> ventilation_withERC_zone9/1
  Product2/1 -> ventilation_withERC_zone9/3
  ventilation_withERC_zone9/1 -> "[S9]"/1
  Constant 3/1 -> ventilation_withERC_zone9/Enable
  AIB10/1 -> ventilation_withERC_zone10/1
  Product3/1 -> ventilation_withERC_zone10/3
  ventilation_withERC_zone10/1 -> "[S10]"/1
  Constant 6/1 -> ventilation_withERC_zone10/Enable
  Constant 8/1 -> Product/1
  Product/1 -> ventilation_withERC_zone7/3
  Constant 4/1 -> Product/2
  Constant 5/1 -> Product1/1
  Constant 2/1 -> Product1/2
  Constant 9/1 -> Product2/1
  Constant 7/1 -> Product2/2
  Constant 12/1 -> Product3/1
  Constant 10/1 -> Product3/2
  AIB6/1 -> ventilation_withERC_zone6/1
  ventilation_withERC_zone6/1 -> "[S6]"/1
  Constant 13/1 -> ventilation_withERC_zone6/Enable
  Constant 15/1 -> Product4/1
  Product4/1 -> ventilation_withERC_zone6/3
  Constant 14/1 -> Product4/2
  AIB5/1 -> ventilation_withERC_zone5/1
  ventilation_withERC_zone5/1 -> "[S5]"/1
  Constant 16/1 -> ventilation_withERC_zone5/Enable
  Constant 18/1 -> Product5/1
  Product5/1 -> ventilation_withERC_zone5/3
  Constant 17/1 -> Product5/2
  AIB4/1 -> ventilation_withERC_zone4/1
  ventilation_withERC_zone4/1 -> "[S4]"/1
  Constant 19/1 -> ventilation_withERC_zone4/Enable
  Constant 21/1 -> Product6/1
  Product6/1 -> ventilation_withERC_zone4/3
  Constant 20/1 -> Product6/2
  AIB3/1 -> ventilation_withERC_zone3/1
  ventilation_withERC_zone3/1 -> "[S3]"/1
  Constant 22/1 -> ventilation_withERC_zone3/Enable
  Constant 24/1 -> Product7/1
  Product7/1 -> ventilation_withERC_zone3/3
  Constant 23/1 -> Product7/2
  AIB2/1 -> ventilation_withERC_zone2/1
  ventilation_withERC_zone2/1 -> "[S2]"/1
  Constant 25/1 -> ventilation_withERC_zone2/Enable
  Constant 27/1 -> Product8/1
  Product8/1 -> ventilation_withERC_zone2/3
  Constant 26/1 -> Product8/2
  AIB1/1 -> ventilation_withERC_zone1/1
  ventilation_withERC_zone1/1 -> "[S1]"/1
  Constant 28/1 -> ventilation_withERC_zone1/Enable
  WDB/1 -> ventilation_withERC_zone3/2, ventilation_withERC_zone1/2, ventilation_withERC_zone2/2, ventilation_withERC_zone4/2, ventilation_withERC_zone5/2, ventilation_withERC_zone6/2, ventilation_withERC_zone8/2, ventilation_withERC_zone9/2, ventilation_withERC_zone10/2, ventilation_withERC_zone7/2
  Constant 30/1 -> Product9/1
  Product9/1 -> ventilation_withERC_zone1/3
  Constant 29/1 -> Product9/2

== system building_EXAMPLE_v1/HVAC window opening ==
  AIB1 : Inport
  AIB2 : Inport  Port=2
  AIB3 : Inport  Port=3
  AIB4 : Inport  Port=4
  AIB5 : Inport  Port=5
  AIB6 : Inport  Port=6
  WDB : Inport  Port=7
  Constant 1 : Constant  Value=hvac.setpoint_opening_window3.values  VectorParams1D=off
  Constant 2 : Constant  Value=hvac.setpoint_opening_window2.values  VectorParams1D=off
  Constant 4 : Constant  Value=hvac.setpoint_opening_window4.values  VectorParams1D=off
  Constant 6 : Constant  Value=hvac.setpoint_opening_window1.values  VectorParams1D=off
  Constant 7 : Constant  Value=hvac.setpoint_opening_window5.values  VectorParams1D=off
  Constant 9 : Constant  Value=hvac.setpoint_opening_window6.values  VectorParams1D=off
  on{,1..5} (6 alike) : Constant
  window opening zone1 : Subsystem
  window opening zone2 : Subsystem
  window opening zone3 : Subsystem
  window opening zone4 : Subsystem
  window opening zone5 : Subsystem
  window opening zone6 : Subsystem
  WindOpen1 : Outport
  WindOpen2 : Outport  Port=2
  WindOpen3 : Outport  Port=3
  WindOpen4 : Outport  Port=4
  WindOpen5 : Outport  Port=5
  WindOpen6 : Outport  Port=6
  wires:
  AIB1/1 -> window opening zone1/2(AIB)
  window opening zone1/1(state) -> WindOpen1/1
  on2/1 -> window opening zone1/Enable
  AIB2/1 -> window opening zone2/2(AIB)
  window opening zone2/1(state) -> WindOpen2/1
  on1/1 -> window opening zone2/Enable
  AIB4/1 -> window opening zone4/2(AIB)
  window opening zone4/1(state) -> WindOpen4/1
  on/1 -> window opening zone4/Enable
  AIB5/1 -> window opening zone5/2(AIB)
  window opening zone5/1(state) -> WindOpen5/1
  on3/1 -> window opening zone5/Enable
  Constant 6/1 -> window opening zone1/1(setpoint)
  AIB6/1 -> window opening zone6/2(AIB)
  window opening zone6/1(state) -> WindOpen6/1
  on4/1 -> window opening zone6/Enable
  Constant 2/1 -> window opening zone2/1(setpoint)
  Constant 4/1 -> window opening zone4/1(setpoint)
  Constant 7/1 -> window opening zone5/1(setpoint)
  Constant 9/1 -> window opening zone6/1(setpoint)
  WDB/1 -> window opening zone6/3(WDB), window opening zone5/3(WDB), window opening zone4/3(WDB), window opening zone3/3(WDB), window opening zone2/3(WDB), window opening zone1/3(WDB)
  AIB3/1 -> window opening zone3/2(AIB)
  window opening zone3/1(state) -> WindOpen3/1
  on5/1 -> window opening zone3/Enable
  Constant 1/1 -> window opening zone3/1(setpoint)

== system building_EXAMPLE_v1/HVAC window shading ==
  WDB : Inport
  Bus Selector : BusSelector  OutputSignals=Solar_Radiation_beam_normal
  Switch : Switch  Criteria=u2 > Threshold  Threshold=hvac.window_1.I_glob
  Switch1 : Switch  Criteria=u2 > Threshold  Threshold=hvac.window_2.I_glob
  Switch2 : Switch  Criteria=u2 > Threshold  Threshold=hvac.window_4.I_glob
  Switch3 : Switch  Criteria=u2 > Threshold  Threshold=hvac.window_5.I_glob
  Switch4 : Switch  Criteria=u2 > Threshold  Threshold=hvac.window_6.I_glob
  Switch5 : Switch  Criteria=u2 > Threshold  Threshold=hvac.window_5.I_glob
  Transfer Fcn (with initial states) : carnotUIBK/HVAC/electrical heater/Transfer Fcn (with initial states)  N=[1]  D="[3600  1]"  X0=0
  Window shading zone 1 : carnot/Load/General/Repeating_Profile  period=hvac.window_1.timevalues(end)  rep_seq_t=hvac.window_1.timevalues(1:end-1)  rep_seq_d=hvac.window_1.timeduration  rep_seq_y=hvac.window_1.values
  Window shading zone 2 : carnot/Load/General/Repeating_Profile  period=hvac.window_2.timevalues(end)  rep_seq_t=hvac.window_2.timevalues(1:end-1)  rep_seq_d=hvac.window_2.timeduration  rep_seq_y=hvac.window_2.values
  Window shading zone 3 : carnot/Load/General/Repeating_Profile  period=hvac.window_3.timevalues(end)  rep_seq_t=hvac.window_3.timevalues(1:end-1)  rep_seq_d=hvac.window_3.timeduration  rep_seq_y=hvac.window_3.values
  Window shading zone 4 : carnot/Load/General/Repeating_Profile  period=hvac.window_4.timevalues(end)  rep_seq_t=hvac.window_4.timevalues(1:end-1)  rep_seq_d=hvac.window_4.timeduration  rep_seq_y=hvac.window_4.values
  Window shading zone 5 : carnot/Load/General/Repeating_Profile  period=hvac.window_5.timevalues(end)  rep_seq_t=hvac.window_5.timevalues(1:end-1)  rep_seq_d=hvac.window_5.timeduration  rep_seq_y=hvac.window_5.values
  Window shading zone 6 : carnot/Load/General/Repeating_Profile  period=hvac.window_6.timevalues(end)  rep_seq_t=hvac.window_6.timevalues(1:end-1)  rep_seq_d=hvac.window_6.timeduration  rep_seq_y=hvac.window_6.values
  no shading : Constant  Value=0
  window 1 : Outport
  window 2 : Outport  Port=2
  window 3 : Outport  Port=3
  window 4 : Outport  Port=4
  window 5 : Outport  Port=5
  window 6 : Outport  Port=6
  wires:
  WDB/1 -> Bus Selector/1
  Switch/1 -> window 1/1
  Window shading zone 1/1 -> Switch/1
  Bus Selector/1 -> Transfer Fcn (with initial states)/1  "<Solar_Radiation_beam_normal>"
  Switch2/1 -> window 4/1
  Window shading zone 4/1 -> Switch2/1
  Switch1/1 -> window 2/1
  Window shading zone 2/1 -> Switch1/1
  Switch3/1 -> window 5/1
  Window shading zone 5/1 -> Switch3/1
  Switch4/1 -> window 6/1
  Window shading zone 6/1 -> Switch4/1
  no shading/1 -> Switch3/3, Switch5/3, Switch/3, Switch1/3, Switch2/3, Switch4/3
  Switch5/1 -> window 3/1
  Window shading zone 3/1 -> Switch5/1
  Transfer Fcn (with initial states)/1 -> Switch5/2, Switch4/2, Switch3/2, Switch2/2, Switch1/2, Switch/2

== system building_EXAMPLE_v1/BUILDING/INTERSECTION_1_10 ==
  AIB1 : Inport
  AIB2 : Inport  Port=2
  BDB1 : Inport  Port=3
  BDB2 : Inport  Port=4
  control : Inport  Port=5
  Add : Sum  Inputs=++++++
  Add1 : Sum  Inputs=++++++
  Bus Selector : BusSelector  OutputSignals=Qdot_S
  Bus Selector1 : BusSelector  OutputSignals=Qdot_S
  airexchange_1 : Subsystem  Variant=on  mask{zone=i.matrix_wd, window=1}
      mask prompts: window "wall"
      mask init:
      | if (window <= size(zone,1))
      |     area = zone{window,2};
      |     height = zone{window,14};
      |     inf_C = zone{window,15};
      |     inf_n = zone{window,16};
      |     inf_V = zone{window,17};
      |     control = zone{window,18};
      | else
      |     area = 0;
      |     height = 0;
      |     inf_C = [0 0 0];
      |     inf_n = [0 0 0];
      |     inf_V = [0 0 0];
      |     control = 1;
      | end
      mask Display:
      | fprintf('AIR EXCHANGE\n')
      | %fprintf('\n%s', const.name)
  airexchange_2 : Subsystem  Variant=on  mask{zone=i.matrix_wd, window=2}
      mask prompts: window "wall"
      mask init: same as building_EXAMPLE_v1/BUILDING/INTERSECTION_1_10/airexchange_1
      mask Display:
      | fprintf('AIR EXCHANGE\n')
      | %fprintf('\n%s', const.name)
  airexchange_3 : Subsystem  Variant=on  mask{zone=i.matrix_wd, window=3}
      mask prompts: window "wall"
      mask init: same as building_EXAMPLE_v1/BUILDING/INTERSECTION_1_10/airexchange_1
      mask Display:
      | fprintf('AIR EXCHANGE\n')
      | %fprintf('\n%s', const.name)
  wall_1 : Subsystem  Variant=on  mask{zone=i.matrix_wd, construction=b.construction, wall=1}
      mask init:
      | if (wall <= size(zone,1))
      |     const = construction.get_structure(zone(wall,1))
      |     wallsurface = zone{wall,2};
      |     pos = [zone{wall,4} zone{wall,5} zone{wall,6}];
      |     view_factor = zone{wall,9};
      |     amb_factor = zone{wall,10};
      |     solar_r = zone{wall,11};
      |     solar_ratio1 = solar_r(1);
      |     solar_ratio2 = solar_r(2);
      |     boundary = zone{wall,12};
      |     % still to be implemented with ENABLE, not a VARIANT!
      |     model_ht = zone{wall,8};
      | else
      |     const.name = 'no construction';
      |     wallsurface = 0;
      |     pos = [0 0 0];
      |     view_factor = 0;
      |     amb_factor = 0;
      |     solar_ratio1 = 0;
      |     solar_ratio2 = 0;
      |     boundary = 0;
      |     model_ht = 0;
      | end
      mask Display:
      | fprintf('CONSTRUCTION:\n')
      | fprintf('\n%s', const.name)
  wall_2 : Subsystem  Variant=on  mask{zone=i.matrix_wd, construction=b.construction, wall=2}
      mask init: same as building_EXAMPLE_v1/BUILDING/INTERSECTION_1_10/wall_1
      mask Display:
      | fprintf('CONSTRUCTION:\n')
      | fprintf('\n%s', const.name)
  wall_3 : Subsystem  Variant=on  mask{zone=i.matrix_wd, construction=b.construction, wall=3}
      mask init: same as building_EXAMPLE_v1/BUILDING/INTERSECTION_1_10/wall_1
      mask Display:
      | fprintf('CONSTRUCTION:\n')
      | fprintf('\n%s', const.name)
  S1 : Outport
  S2 : Outport  Port=2
  wires:
  Add/1 -> S1/1
  Add1/1 -> S2/1
  BDB1/1 -> Bus Selector/1
  Bus Selector/1 -> wall_1/3(Qdot_sol1), wall_2/3(Qdot_sol1), wall_3/3(Qdot_sol1)  "<Qdot_S>"
  BDB2/1 -> Bus Selector1/1
  Bus Selector1/1 -> wall_1/4(Qdot_sol2), wall_2/4(Qdot_sol2), wall_3/4(Qdot_sol2)  "<Qdot_S>"
  control/1 -> airexchange_3/3(control), airexchange_2/3(control), airexchange_1/3(control)
  AIB2/1 -> wall_2/2(AIB2), wall_3/2(AIB2), airexchange_3/2(AIB2), airexchange_2/2(AIB2), airexchange_1/2(AIB2), wall_1/2(AIB2)
  AIB1/1 -> wall_2/1(AIB1), wall_3/1(AIB1), airexchange_3/1(AIB1), airexchange_2/1(AIB1), airexchange_1/1(AIB1), wall_1/1(AIB1)
  wall_1/1("[S1]") -> Add/1
  wall_2/1("[S1]") -> Add/2
  wall_3/1("[S1]") -> Add/3
  airexchange_1/1("[S1]") -> Add/4
  airexchange_2/1("[S1]") -> Add/5
  airexchange_3/1("[S1]") -> Add/6
  wall_1/2("[S2]") -> Add1/1
  wall_2/2("[S2]") -> Add1/2
  airexchange_3/2("[S2]") -> Add1/6
  airexchange_2/2("[S2]") -> Add1/5
  airexchange_1/2("[S2]") -> Add1/4
  wall_3/2("[S2]") -> Add1/3

== system building_EXAMPLE_v1/BUILDING/INTERSECTION_1_2 ==
  AIB1 : Inport
  AIB2 : Inport  Port=2
  BDB1 : Inport  Port=3
  BDB2 : Inport  Port=4
  control : Inport  Port=5
  Add : Sum  Inputs=++++++
  Add1 : Sum  Inputs=++++++
  Bus Selector : BusSelector  OutputSignals=Qdot_S
  Bus Selector1 : BusSelector  OutputSignals=Qdot_S
  airexchange_1 : Subsystem  Variant=on  mask{zone=i.matrix_wd, window=1}
      mask prompts: window "wall"
      mask init: same as building_EXAMPLE_v1/BUILDING/INTERSECTION_1_10/airexchange_1
      mask Display:
      | fprintf('AIR EXCHANGE\n')
      | %fprintf('\n%s', const.name)
  airexchange_2 : Subsystem  Variant=on  mask{zone=i.matrix_wd, window=2}
      mask prompts: window "wall"
      mask init: same as building_EXAMPLE_v1/BUILDING/INTERSECTION_1_10/airexchange_1
      mask Display:
      | fprintf('AIR EXCHANGE\n')
      | %fprintf('\n%s', const.name)
  airexchange_3 : Subsystem  Variant=on  mask{zone=i.matrix_wd, window=3}
      mask prompts: window "wall"
      mask init: same as building_EXAMPLE_v1/BUILDING/INTERSECTION_1_10/airexchange_1
      mask Display:
      | fprintf('AIR EXCHANGE\n')
      | %fprintf('\n%s', const.name)
  wall_1 : Subsystem  Variant=on  mask{zone=i.matrix_wd, construction=b.construction, wall=1}
      mask init: same as building_EXAMPLE_v1/BUILDING/INTERSECTION_1_10/wall_1
      mask Display:
      | fprintf('CONSTRUCTION:\n')
      | fprintf('\n%s', const.name)
  wall_2 : Subsystem  Variant=on  mask{zone=i.matrix_wd, construction=b.construction, wall=2}
      mask init: same as building_EXAMPLE_v1/BUILDING/INTERSECTION_1_10/wall_1
      mask Display:
      | fprintf('CONSTRUCTION:\n')
      | fprintf('\n%s', const.name)
  wall_3 : Subsystem  Variant=on  mask{zone=i.matrix_wd, construction=b.construction, wall=3}
      mask init: same as building_EXAMPLE_v1/BUILDING/INTERSECTION_1_10/wall_1
      mask Display:
      | fprintf('CONSTRUCTION:\n')
      | fprintf('\n%s', const.name)
  S1 : Outport
  S2 : Outport  Port=2
  wires:
  Add/1 -> S1/1
  Add1/1 -> S2/1
  BDB1/1 -> Bus Selector/1
  Bus Selector/1 -> wall_1/3(Qdot_sol1), wall_2/3(Qdot_sol1), wall_3/3(Qdot_sol1)  "<Qdot_S>"
  BDB2/1 -> Bus Selector1/1
  Bus Selector1/1 -> wall_1/4(Qdot_sol2), wall_2/4(Qdot_sol2), wall_3/4(Qdot_sol2)  "<Qdot_S>"
  control/1 -> airexchange_3/3(control), airexchange_2/3(control), airexchange_1/3(control)
  AIB2/1 -> wall_2/2(AIB2), wall_3/2(AIB2), airexchange_3/2(AIB2), airexchange_2/2(AIB2), airexchange_1/2(AIB2), wall_1/2(AIB2)
  AIB1/1 -> wall_2/1(AIB1), wall_3/1(AIB1), airexchange_3/1(AIB1), airexchange_2/1(AIB1), airexchange_1/1(AIB1), wall_1/1(AIB1)
  wall_1/1("[S1]") -> Add/1
  wall_2/1("[S1]") -> Add/2
  wall_3/1("[S1]") -> Add/3
  airexchange_1/1("[S1]") -> Add/4
  airexchange_2/1("[S1]") -> Add/5
  airexchange_3/1("[S1]") -> Add/6
  wall_1/2("[S2]") -> Add1/1
  wall_2/2("[S2]") -> Add1/2
  airexchange_3/2("[S2]") -> Add1/6
  airexchange_2/2("[S2]") -> Add1/5
  airexchange_1/2("[S2]") -> Add1/4
  wall_3/2("[S2]") -> Add1/3
